simulink model "KP_Nikolaev_v8"  (R2021a)
settings: Solver=VariableStepAuto  StartTime=0.0  StopTime=30  RelTol=0.05
undefined symbols (not defined in the file): D11, Delta
libraries: spsThreePhaseBreakerLib x35, spsSeriesRLCBranchLib x24, spsThreePhaseSeriesRLCLoadLib x22, slrealtimeutilitieslib x14, slrealtimeiplib x13, spsThreePhaseVIMeasurementLib x8, spsExcitationSystemLib x3, spsSynchronousMachinepuStandardLib x3, spsSteamTurbineandGovernorLib x2, spsThreePhaseTransformerTwoWindingsLib x2, spsGroundLib x1, spsHydraulicTurbineandGovernorLib x1
settings Model: Creator=kirill  LastModifiedBy=1
settings SolverCC: AlgebraicLoopSolver=TrustRegion
settings DebuggingCC: UnconnectedInputMsg=none  UnconnectedOutputMsg=none  UnconnectedLineMsg=none  SFMachineParentedDataDiag=warning

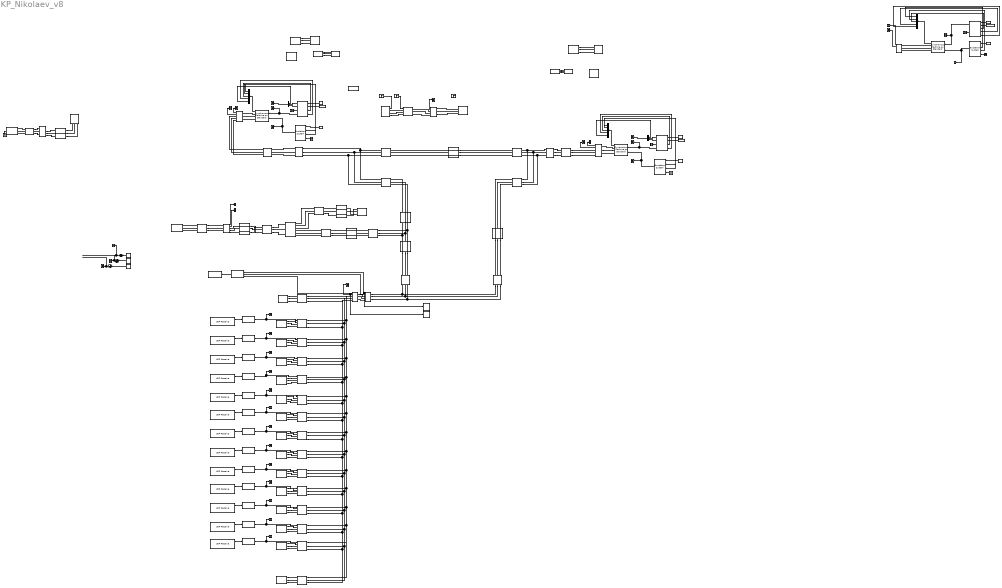
== system KP_Nikolaev_v8 ==
  Breaker0 : spsThreePhaseBreakerLib/Three-Phase Breaker  InitialState=open  SwitchA=on  SwitchB=on  SwitchC=on  SwitchTimes="[1/60  5/60]"  External=off  BreakerResistance=0.01  SnubberResistance=1e6  SnubberCapacitance=inf  Measurements=None
  Breaker{1..13,34} (14 alike) : spsThreePhaseBreakerLib/Three-Phase Breaker  InitialState=closed  SwitchA=on  SwitchB=on  SwitchC=on  SwitchTimes="[1/60  5/60]"  External=on  BreakerResistance=0.01  SnubberResistance=1e6  SnubberCapacitance=inf  Measurements=None
  Breaker{14..32} (19 alike) : spsThreePhaseBreakerLib/Three-Phase Breaker  InitialState=closed  SwitchA=on  SwitchB=on  SwitchC=on  SwitchTimes="[1/60  5/60]"  External=off  BreakerResistance=0.01  SnubberResistance=1e6  SnubberCapacitance=inf  Measurements=None
  Breaker33 : spsThreePhaseBreakerLib/Three-Phase Breaker  InitialState=open  SwitchA=on  SwitchB=on  SwitchC=on  SwitchTimes="[1/60  5/60]"  External=on  BreakerResistance=0.01  SnubberResistance=1e6  SnubberCapacitance=inf  Measurements=None
  Bus Creator1 : BusCreator  Inputs=3
  Bus Creator2 : BusCreator  Inputs=3
  Bus Selector1 : BusSelector  OutputSignals="dq0 components.Stator voltage  vd (pu),dq0 components.Stator voltage  vq (pu),Mechanical.Rotor speed  wm  (pu),Mechanical.Rotor angle deviation  d_theta (rad),Mechanical.Rotor speed deviation  dw (pu)"
  Bus Selector2 : BusSelector  OutputSignals="dq0 components.Stator voltage  vd (pu),dq0 components.Stator voltage  vq (pu),Mechanical.Rotor speed  wm  (pu),Mechanical.Rotor angle deviation  d_theta (rad),Mechanical.Rotor speed deviation  dw (pu)"
  Bus Selector3 : BusSelector  OutputSignals="dq0 components.Stator voltage  vd (pu),dq0 components.Stator voltage  vq (pu),Mechanical.Rotor speed  wm  (pu),Output active power   Peo (pu),Mechanical.Rotor speed deviation  dw (pu)"
  Byte Packing : slrealtimeutilitieslib/Byte Packing  MaskPackedDataType=double  MaskUnpackedDataTypes={'double' 'double' 'double'}  MaskAlignment=1
  Byte Unpacking{,1..11,13} (13 alike) : slrealtimeutilitieslib/Byte Unpacking  MaskUnpackedDataTypes={'double'}  MaskUnpackedDataSizes={[1]}  MaskAlignment=1
      settings: SourceProductBaseCode=XP
  Constant{,1..2,4..5,8} (6 alike) : Constant
  Constant3 : Constant  Value=0.151964
  Constant6 : Constant  Value=0.151964
  Constant7 : Constant  Value=0.90671
  Excitation System : spsExcitationSystemLib/Excitation System  tr=10e-4  reg=[ 200, 0.001 ]  exc=[ 5, 0 ]  tgr=[ 0, 0 ]  damp=[ 0.001, 0.1 ]  sat=[ 0, 0 ]  lim=[ -15, 15, 0 ]  v0=[1,2.93164]
      settings: SourceProductBaseCode=PS
  Excitation System1 : spsExcitationSystemLib/Excitation System  tr=10e-3  reg=[ 19, 0.001 ]  exc=[ 3, 0 ]  tgr=[ 0, 0 ]  damp=[ 0.001, 0.1 ]  sat=[ 0, 0 ]  lim=[ -11.5, 11.5, 0 ]  v0=[1,1.07632]
      settings: SourceProductBaseCode=PS
  Excitation System2 : spsExcitationSystemLib/Excitation System  tr=10e-3  reg=[ 19, 0.001 ]  exc=[ 3, 0 ]  tgr=[ 0, 0 ]  damp=[ 0.001, 0.1 ]  sat=[ 0, 0 ]  lim=[ -11.5, 11.5, 0 ]  v0=[1,1.07632]
      settings: SourceProductBaseCode=PS
  Ground : Ground
  Ground1 : Ground
  Ground2 : Ground
  Ground3 : spsGroundLib/Ground  LConnTagsString=a
  HTG1 : spsHydraulicTurbineandGovernorLib/Hydraulic Turbine and Governor  sm="[ 1  0.77 ]"  gate="[  0.01  0.97518  -0.1  0.1 ]"  reg="[  0.1  0.090 0.005 0.001  1  ]"  hyd="[  0  2.67  ]"  dref=0  po=0.946226
      settings: SourceProductBaseCode=PS
  Scope{1..34} (34 alike) : Scope
  Series RLC Branch{1..3,18..20} (6 alike) : spsSeriesRLCBranchLib/Series RLC Branch  LConnTagsString=__new0  RConnTagsString=__new0  BranchType=RLC  Resistance=12.45  Inductance=70.187e-3  SetiL0=off  InitialCurrent=0  Capacitance=4.07436e-3  Setx0=off  InitialVoltage=0  Measurements=None
  Series RLC Branch{4..6,9..11} (6 alike) : spsSeriesRLCBranchLib/Series RLC Branch  LConnTagsString=__new0  RConnTagsString=__new0  BranchType=RLC  Resistance=6.225  Inductance=35.0935e-3  SetiL0=off  InitialCurrent=0  Capacitance=2.03718e-3  Setx0=off  InitialVoltage=0  Measurements=None
  Series RLC Branch12 : spsSeriesRLCBranchLib/Series RLC Branch  LConnTagsString=__new0  RConnTagsString=__new0  BranchType=RLC  Resistance=9.75  Inductance=70e-3  SetiL0=off  InitialCurrent=0  Capacitance=4.07436e-3  Setx0=off  InitialVoltage=0  Measurements=None
  Series RLC Branch{8,13..14,21} (4 alike) : spsSeriesRLCBranchLib/Series RLC Branch  LConnTagsString=__new0  RConnTagsString=__new0  BranchType=RLC  Resistance=9.75  Inductance=70e-3  SetiL0=off  InitialCurrent=0  Capacitance=4e-3  Setx0=off  InitialVoltage=0  Measurements=None
  Series RLC Branch15 : spsSeriesRLCBranchLib/Series RLC Branch  LConnTagsString=__new0  RConnTagsString=__new0  BranchType=RLC  Resistance=9.25  Inductance=70.187e-3  SetiL0=off  InitialCurrent=0  Capacitance=4.07436e-3  Setx0=off  InitialVoltage=0  Measurements=None
  Series RLC Branch16 : spsSeriesRLCBranchLib/Series RLC Branch  LConnTagsString=__new0  RConnTagsString=__new0  BranchType=RLC  Resistance=9.25  Inductance=70.187e-3  SetiL0=off  InitialCurrent=0  Capacitance=4.07436e-3  Setx0=off  InitialVoltage=0  Measurements=None
  Series RLC Branch17 : spsSeriesRLCBranchLib/Series RLC Branch  LConnTagsString=__new0  RConnTagsString=__new0  BranchType=RLC  Resistance=9.25  Inductance=70.187e-3  SetiL0=off  InitialCurrent=0  Capacitance=4.07436e-3  Setx0=off  InitialVoltage=0  Measurements=None
  Series RLC Branch22 : spsSeriesRLCBranchLib/Series RLC Branch  LConnTagsString=__new0  RConnTagsString=__new0  BranchType=RLC  Resistance=19.5  Inductance=70e-3  SetiL0=off  InitialCurrent=0  Capacitance=4.07436e-3  Setx0=off  InitialVoltage=0  Measurements=None
  Series RLC Branch23 : spsSeriesRLCBranchLib/Series RLC Branch  LConnTagsString=__new0  RConnTagsString=__new0  BranchType=RLC  Resistance=19.5  Inductance=70e-3  SetiL0=off  InitialCurrent=0  Capacitance=4e-3  Setx0=off  InitialVoltage=0  Measurements=None
  Series RLC Branch24 : spsSeriesRLCBranchLib/Series RLC Branch  LConnTagsString=__new0  RConnTagsString=__new0  BranchType=RLC  Resistance=19.5  Inductance=70e-3  SetiL0=off  InitialCurrent=0  Capacitance=4e-3  Setx0=off  InitialVoltage=0  Measurements=None
  Series RLC Branch7 : spsSeriesRLCBranchLib/Series RLC Branch  LConnTagsString=__new0  RConnTagsString=__new0  BranchType=RLC  Resistance=9.75  Inductance=70e-3  SetiL0=off  InitialCurrent=0  Capacitance=4.07436e-3  Setx0=off  InitialVoltage=0  Measurements=None
  Spectrum Analyzer : SpectrumAnalyzer
  Spectrum Analyzer1 : SpectrumAnalyzer
  Steam Turbine and Governor1 : spsSteamTurbineandGovernorLib/Steam Turbine and Governor  gentype=Tandem-compound (single mass)  reg1="[ 5 0.05  0 ]"  reg2="[ 0.001  0.15 ]"  reg3="[ -0.1 0.1  0  10.496]"  N=3000  turb1="[ 0  40 20  2 ]"  turb2="[ 0.5   0.5   0.0  0 ]"  HA="[  1.5498   0.24894  0  0 ]"  KA="[  83.47  42.702  0  0 ]"  DA="[  0.3104  0.05  0  0 ]*8"  ini1=0.173417  ini2=[0.429327,-63.9543]
      settings: SourceProductBaseCode=PS
  Steam Turbine and Governor2 : spsSteamTurbineandGovernorLib/Steam Turbine and Governor  gentype=Tandem-compound (single mass)  reg1="[ 5 0.05  0 ]"  reg2="[ 0.001  0.15 ]"  reg3="[ -0.1 0.1  0  10.496]"  N=3000  turb1="[ 0  40 20  2 ]"  turb2="[ 0.5   0.5   0.0  0 ]"  HA="[  1.5498   0.24894  0  0 ]"  KA="[  83.47  42.702  0  0 ]"  DA="[  0.3104  0.05  0  0 ]*8"  ini1=0.173417  ini2=[0.429327,-63.9543]
      settings: SourceProductBaseCode=PS
  Step : Step  Time=5  SampleTime=0  VectorParams1D=off
  Step1 : Step  Time=7  Before=1  After=0  SampleTime=0  VectorParams1D=off
  Step2 : Step  Time=5  SampleTime=0  VectorParams1D=off
  Sum : Sum  Inputs=|++
  Sum1 : Sum  Inputs=|++
  Sum2 : Sum  Inputs=|++
  Synchronous Machine : spsSynchronousMachinepuStandardLib/Synchronous Machine pu Standard  PresetModel=No  MechanicalLoad=Mechanical power Pm  ShowDetailedParameters=on  RotorType=Salient-pole  Units=per unit standard parameters  MeasurementBus=off  NominalParameters=[25.88e+06 9.785e+03 50]  Reactances1=[ 1.81, 0.3, 0.23, 1.76, 0.65, 0.25, 0.15 ]  Reactances2=[0.8 0.35 0.22 0.59 0.23 0.1]  dAxisTimeConstants=Short-circuit  qAxisTimeConstants=Short-circuit  TimeConstants1="[ 4.4849  0.0681  0.1  ]"  TimeConstants2=[ 8.0, 0.03, 1.0, 0.07 ]  TimeConstants3="[  4.49  0.0681  0.0513  ]"  TimeConstants4=[ 8.0, 0.03, 0.3371, 0.0295 ]  TimeConstants5=[ 1.01, 0.053, 0.1 ]  TimeConstants6=[ 1.3201, 0.023, 1.0, 0.07 ]  TimeConstants7=[0.012 0.003 0.003]  TimeConstants8=[ 1.3201, 0.0231, 0.3371, 0.0295 ]  StatorResistance=0.037875  Mechanical=[0.1028 0.02056 52]  PolePairs=20  InitialConditions=[0 -53.0957 3.14495 3.14495 3.14495 -25.3073 -145.307 94.6927 2.93164]  SetSaturation=on  Saturation=[0.6404,0.7127,0.8441,0.9214,0.9956,1.082,1.19,1.316,1.457;0.7,0.7698,0.8872,0.9466,0.9969,1.046,1.1,1.151,1.201]  LoadFlowParameters=[2 107000000 0 0 0]  TsPowergui=0  TsBlock=-1  IterativeModel=Trapezoidal non iterative  IterativeDiscreteModel=Trapezoidal robust  BusType=swing  Pref=109.0152  Qref=62.94  Qmin=-Inf  Qmax=Inf  PLF=0  QLF=0
      settings: SourceProductBaseCode=PS
  Synchronous Machine1 : spsSynchronousMachinepuStandardLib/Synchronous Machine pu Standard  PresetModel=No  MechanicalLoad=Mechanical power Pm  ShowDetailedParameters=on  RotorType=Round  Units=per unit standard parameters  MeasurementBus=off  NominalParameters=[78.75e+06 7.424e+03 50]  Reactances1=[ 1.915, 0.275, 0.203, 0.82, 0.65, 0.25, 0.15 ]  Reactances2=[1.71 0.172 0.119 0.59 0.23 0.1]  dAxisTimeConstants=Short-circuit  qAxisTimeConstants=Short-circuit  TimeConstants1="[ 4.4849  0.0681  0.1  ]"  TimeConstants2=[ 8.0, 0.03, 1.0, 0.07 ]  TimeConstants3="[  4.49  0.0681  0.0513  ]"  TimeConstants4=[ 8.0, 0.03, 0.3371, 0.0295 ]  TimeConstants5=[ 1.01, 0.053, 0.1 ]  TimeConstants6=[ 1.3201, 0.023, 1.0, 0.07 ]  TimeConstants7=[1.42 0.0908 0.132]  TimeConstants8=[ 1.85, 0.126, 0.212, 0.169 ]  StatorResistance=0.037875  Mechanical=[0.1028 0.02056 1]  PolePairs=20  InitialConditions=[0 -99.9478 0.153639 0.153639 0.153639 -25.3073 -145.307 94.6927 1.07632]  SetSaturation=on  Saturation=[0.6404,0.7127,0.8441,0.9214,0.9956,1.082,1.19,1.316,1.457;0.7,0.7698,0.8872,0.9466,0.9969,1.046,1.1,1.151,1.201]  LoadFlowParameters=[2 7500000 0 0 0]  TsPowergui=0  TsBlock=-1  IterativeModel=Trapezoidal non iterative  IterativeDiscreteModel=Trapezoidal robust  BusType=swing  Pref=2e+06  Qref=1e+06  Qmin=-Inf  Qmax=Inf  PLF=0  QLF=0
      settings: SourceProductBaseCode=PS
  Synchronous Machine2 : spsSynchronousMachinepuStandardLib/Synchronous Machine pu Standard  PresetModel=No  MechanicalLoad=Mechanical power Pm  ShowDetailedParameters=on  RotorType=Round  Units=per unit standard parameters  MeasurementBus=off  NominalParameters=[78.75e+06 7.424e+03 50]  Reactances1=[ 1.915, 0.275, 0.203, 0.82, 0.65, 0.25, 0.15 ]  Reactances2=[1.71 0.172 0.119 0.59 0.23 0.1]  dAxisTimeConstants=Short-circuit  qAxisTimeConstants=Short-circuit  TimeConstants1="[ 4.4849  0.0681  0.1  ]"  TimeConstants2=[ 8.0, 0.03, 1.0, 0.07 ]  TimeConstants3="[  4.49  0.0681  0.0513  ]"  TimeConstants4=[ 8.0, 0.03, 0.3371, 0.0295 ]  TimeConstants5=[ 1.01, 0.053, 0.1 ]  TimeConstants6=[ 1.3201, 0.023, 1.0, 0.07 ]  TimeConstants7=[1.42 0.0908 0.132]  TimeConstants8=[ 1.85, 0.126, 0.212, 0.169 ]  StatorResistance=0.037875  Mechanical=[0.1028 0.02056 1]  PolePairs=20  InitialConditions=[0 -99.9478 0.153639 0.153639 0.153639 -25.3073 -145.307 94.6927 1.07632]  SetSaturation=on  Saturation=[0.6404,0.7127,0.8441,0.9214,0.9956,1.082,1.19,1.316,1.457;0.7,0.7698,0.8872,0.9466,0.9969,1.046,1.1,1.151,1.201]  LoadFlowParameters=[2 7500000 0 0 0]  TsPowergui=0  TsBlock=-1  IterativeModel=Trapezoidal non iterative  IterativeDiscreteModel=Trapezoidal robust  BusType=swing  Pref=2e+06  Qref=1e+06  Qmin=-Inf  Qmax=Inf  PLF=0  QLF=0
      settings: SourceProductBaseCode=PS
  T1 : spsThreePhaseTransformerInductanceMatrixTypeThreeWindingsLib/Three-Phase Transformer Inductance Matrix Type (Three Windings)  CoreType=Three single-phase cores  Winding1Connection=Y  Winding2Connection=Delta (D11)  Winding3Connection=Delta (D11)  AutoTransformer=off  Measurements=None  NominalPower="[133e6,  50]"  VLLnom="[330e3,  230e3,  38.5e3]"  WindingResistances="[0.005,  0.005, 0.005]"  NoLoadIexcPos=0.06  NoLoadPlossPos=50e3  ShortCircuitReactancePos="[0.087,  0.166,  0.067]"  ShortCircuitReactancePosAuto="[0.087,  0.166,  0.067]"  NoLoadIexcZero=100  NoLoadPlossZero=133e6*1/100  ShortCircuitReactanceZero=[0.1, 0.2, 0.3 ]  ShortCircuitReactanceZeroAuto=[0.1, 0.2, 0.3 ]  X12ZeroMeasuredWithW3Delta=off
      settings: SourceProductBaseCode=PS
  Terminator : Terminator
  Terminator1 : Terminator
  Terminator2 : Terminator
  Three-Phase Measurement 1 : spsThreePhaseVIMeasurementLib/Three-Phase V-I Measurement  VoltageMeasurement=phase-to-ground  SetLabelV=off  LabelV=Vabc  Vpu=off  VpuLL=off  CurrentMeasurement=yes  SetLabelI=off  LabelI=Iabc  Ipu=off  Pbase=100e6  Vbase=115e3  OutputType=Complex  PhasorSimulation=off  PSBequivalent=0
  Three-Phase Measurement 2 : spsThreePhaseVIMeasurementLib/Three-Phase V-I Measurement  VoltageMeasurement=phase-to-phase  SetLabelV=off  LabelV=Vabc  Vpu=off  VpuLL=off  CurrentMeasurement=yes  SetLabelI=off  LabelI=Iabc  Ipu=off  Pbase=100e6  Vbase=500e3  OutputType=Complex  PhasorSimulation=off  PSBequivalent=0
  Three-Phase Measurement 4 : spsThreePhaseVIMeasurementLib/Three-Phase V-I Measurement  VoltageMeasurement=phase-to-ground  SetLabelV=off  LabelV=Vabc  Vpu=off  VpuLL=off  CurrentMeasurement=yes  SetLabelI=off  LabelI=Iabc  Ipu=off  Pbase=100e6  Vbase=115e3  OutputType=Complex  PhasorSimulation=off  PSBequivalent=0
  Three-Phase Measurement 9 : spsThreePhaseVIMeasurementLib/Three-Phase V-I Measurement  VoltageMeasurement=phase-to-phase  SetLabelV=off  LabelV=Vabc  Vpu=off  VpuLL=off  CurrentMeasurement=yes  SetLabelI=off  LabelI=Iabc  Ipu=off  Pbase=100e6  Vbase=500e3  OutputType=Complex  PhasorSimulation=off  PSBequivalent=0
  Three-Phase RL Load0 : spsThreePhaseSeriesRLCLoadLib/Three-Phase Series RLC Load  LConnTagsString=A|B|C  Configuration=Y (grounded)  NominalVoltage=230000  Vabc=[1e3 1e3 1e3]  Vabcp=[1e3 1e3 1e3]  NominalFrequency=50  UnbalancedPower=off  ActivePower=78.5225e+06  InductivePower=33.4873e+06  CapacitivePower=500  Pabc=[10e3 9e3 11e3]  QLabc=[100 90 110]  QCabc=[100 90 110]  Pabcp=[10e3 9e3 11e3]  QLabcp=[100 90 110]  QCabcp=[100 90 110]  Measurements=None  LoadType=constant PQ
  Three-Phase RL Load{1..11} (11 alike) : spsThreePhaseSeriesRLCLoadLib/Three-Phase Series RLC Load  LConnTagsString=A|B|C  Configuration=Y (grounded)  NominalVoltage=230000  Vabc=[1e3 1e3 1e3]  Vabcp=[1e3 1e3 1e3]  NominalFrequency=50  UnbalancedPower=off  ActivePower=8.144e+06  InductivePower=3.47264e+06  CapacitivePower=50  Pabc=[10e3 9e3 11e3]  QLabc=[100 90 110]  QCabc=[100 90 110]  Pabcp=[10e3 9e3 11e3]  QLabcp=[100 90 110]  QCabcp=[100 90 110]  Measurements=None  LoadType=constant PQ
  Three-Phase RL Load12 : spsThreePhaseSeriesRLCLoadLib/Three-Phase Series RLC Load  LConnTagsString=A|B|C  Configuration=Y (grounded)  NominalVoltage=230000  Vabc=[1e3 1e3 1e3]  Vabcp=[1e3 1e3 1e3]  NominalFrequency=50  UnbalancedPower=off  ActivePower=17.948e+06  InductivePower=7.6532e+06  CapacitivePower=100  Pabc=[10e3 9e3 11e3]  QLabc=[100 90 110]  QCabc=[100 90 110]  Pabcp=[10e3 9e3 11e3]  QLabcp=[100 90 110]  QCabcp=[100 90 110]  Measurements=None  LoadType=constant PQ
  Three-Phase RL Load13 : spsThreePhaseSeriesRLCLoadLib/Three-Phase Series RLC Load  LConnTagsString=A|B|C  Configuration=Y (grounded)  NominalVoltage=230000  Vabc=[1e3 1e3 1e3]  Vabcp=[1e3 1e3 1e3]  NominalFrequency=50  UnbalancedPower=off  ActivePower=17.948e+06  InductivePower=7.6532e+06  CapacitivePower=100  Pabc=[10e3 9e3 11e3]  QLabc=[100 90 110]  QCabc=[100 90 110]  Pabcp=[10e3 9e3 11e3]  QLabcp=[100 90 110]  QCabcp=[100 90 110]  Measurements=None  LoadType=constant PQ
  Three-Phase RL Load14 : spsThreePhaseSeriesRLCLoadLib/Three-Phase Series RLC Load  LConnTagsString=A|B|C  Configuration=Y (grounded)  NominalVoltage=10500  Vabc=[1e3 1e3 1e3]  Vabcp=[1e3 1e3 1e3]  NominalFrequency=50  UnbalancedPower=off  ActivePower=4500  InductivePower=0  CapacitivePower=0  Pabc=[10e3 9e3 11e3]  QLabc=[100 90 110]  QCabc=[100 90 110]  Pabcp=[10e3 9e3 11e3]  QLabcp=[100 90 110]  QCabcp=[100 90 110]  Measurements=None  LoadType=constant PQ
  Three-Phase RL Load15 : spsThreePhaseSeriesRLCLoadLib/Three-Phase Series RLC Load  LConnTagsString=A|B|C  Configuration=Y (grounded)  NominalVoltage=230000  Vabc=[1e3 1e3 1e3]  Vabcp=[1e3 1e3 1e3]  NominalFrequency=50  UnbalancedPower=off  ActivePower=98.714e+06  InductivePower=42.0926e+06  CapacitivePower=1000  Pabc=[10e3 9e3 11e3]  QLabc=[100 90 110]  QCabc=[100 90 110]  Pabcp=[10e3 9e3 11e3]  QLabcp=[100 90 110]  QCabcp=[100 90 110]  Measurements=None  LoadType=constant PQ
  Three-Phase RL Load16 : spsThreePhaseSeriesRLCLoadLib/Three-Phase Series RLC Load  LConnTagsString=A|B|C  Configuration=Y (grounded)  NominalVoltage=10500  Vabc=[1e3 1e3 1e3]  Vabcp=[1e3 1e3 1e3]  NominalFrequency=50  UnbalancedPower=off  ActivePower=4500  InductivePower=0  CapacitivePower=0  Pabc=[10e3 9e3 11e3]  QLabc=[100 90 110]  QCabc=[100 90 110]  Pabcp=[10e3 9e3 11e3]  QLabcp=[100 90 110]  QCabcp=[100 90 110]  Measurements=None  LoadType=constant PQ
  Three-Phase RL Load17 : spsThreePhaseSeriesRLCLoadLib/Three-Phase Series RLC Load  LConnTagsString=A|B|C  Configuration=Y (grounded)  NominalVoltage=10500  Vabc=[1e3 1e3 1e3]  Vabcp=[1e3 1e3 1e3]  NominalFrequency=50  UnbalancedPower=off  ActivePower=1.75e+06  InductivePower=1e+06  CapacitivePower=100  Pabc=[10e3 9e3 11e3]  QLabc=[100 90 110]  QCabc=[100 90 110]  Pabcp=[10e3 9e3 11e3]  QLabcp=[100 90 110]  QCabcp=[100 90 110]  Measurements=None  LoadType=constant PQ
  Three-Phase RL Load18 : spsThreePhaseSeriesRLCLoadLib/Three-Phase Series RLC Load  LConnTagsString=A|B|C  Configuration=Y (grounded)  NominalVoltage=10500  Vabc=[1e3 1e3 1e3]  Vabcp=[1e3 1e3 1e3]  NominalFrequency=50  UnbalancedPower=off  ActivePower=3.25e+06  InductivePower=1.875e+06  CapacitivePower=100  Pabc=[10e3 9e3 11e3]  QLabc=[100 90 110]  QCabc=[100 90 110]  Pabcp=[10e3 9e3 11e3]  QLabcp=[100 90 110]  QCabcp=[100 90 110]  Measurements=None  LoadType=constant PQ
  Three-Phase RL Load19 : spsThreePhaseSeriesRLCLoadLib/Three-Phase Series RLC Load  LConnTagsString=A|B|C  Configuration=Y (grounded)  NominalVoltage=10500  Vabc=[1e3 1e3 1e3]  Vabcp=[1e3 1e3 1e3]  NominalFrequency=50  UnbalancedPower=off  ActivePower=1.75e+06  InductivePower=1e+06  CapacitivePower=100  Pabc=[10e3 9e3 11e3]  QLabc=[100 90 110]  QCabc=[100 90 110]  Pabcp=[10e3 9e3 11e3]  QLabcp=[100 90 110]  QCabcp=[100 90 110]  Measurements=None  LoadType=constant PQ
  Three-Phase RL Load20 : spsThreePhaseSeriesRLCLoadLib/Three-Phase Series RLC Load  LConnTagsString=A|B|C  Configuration=Y (grounded)  NominalVoltage=10500  Vabc=[1e3 1e3 1e3]  Vabcp=[1e3 1e3 1e3]  NominalFrequency=50  UnbalancedPower=off  ActivePower=3.25e+06  InductivePower=1.875e+06  CapacitivePower=100  Pabc=[10e3 9e3 11e3]  QLabc=[100 90 110]  QCabc=[100 90 110]  Pabcp=[10e3 9e3 11e3]  QLabcp=[100 90 110]  QCabcp=[100 90 110]  Measurements=None  LoadType=constant PQ
  Three-Phase RL Load21 : spsThreePhaseSeriesRLCLoadLib/Three-Phase Series RLC Load  LConnTagsString=A|B|C  Configuration=Y (grounded)  NominalVoltage=38.5e3  Vabc=[1e3 1e3 1e3]  Vabcp=[1e3 1e3 1e3]  NominalFrequency=50  UnbalancedPower=off  ActivePower=13.65e+06  InductivePower=7.875e+06  CapacitivePower=100  Pabc=[10e3 9e3 11e3]  QLabc=[100 90 110]  QCabc=[100 90 110]  Pabcp=[10e3 9e3 11e3]  QLabcp=[100 90 110]  QCabcp=[100 90 110]  Measurements=None  LoadType=constant PQ
  Three-Phase Transformer (Two Windings)1 : spsThreePhaseTransformerTwoWindingsLib/Three-Phase Transformer (Two Windings)  Winding1Connection=Y  Winding2Connection=Delta (D11)  CoreType=Three single-phase transformers  SetSaturation=off  Hysteresis=off  DataFile='hysteresis'  SetInitialFlux=off  Measurements=None  UNITS=SI  NominalPower=[ 80e6 , 50 ]  Winding1=[10500 0.00882 0.001123]  Winding2=[2.42e+05 11.616 1.479]  Rm=2205  Lm=7.0187  L0=0.5  Saturation=[0 0;4.6657 32.747;1944 41.48]  InitialFluxes=[ 0.8 , -0.8 , 0.7 ]  BreakLoop=on  DiscreteSolver=Trapezoidal iterative  DataType=on  TransfoNumber=1
  Three-Phase Transformer (Two Windings)2 : spsThreePhaseTransformerTwoWindingsLib/Three-Phase Transformer (Two Windings)  Winding1Connection=Y  Winding2Connection=Delta (D11)  CoreType=Three single-phase transformers  SetSaturation=off  Hysteresis=off  DataFile='hysteresis'  SetInitialFlux=off  Measurements=None  UNITS=SI  NominalPower=[ 80e6 , 50 ]  Winding1=[10500 0.00882 0.001123]  Winding2=[2.42e+05 11.616 1.479]  Rm=2205  Lm=7.0187  L0=0.5  Saturation=[0 0;4.6657 32.747;1944 41.48]  InitialFluxes=[ 0.8 , -0.8 , 0.7 ]  BreakLoop=on  DiscreteSolver=Trapezoidal iterative  DataType=on  TransfoNumber=1
  Three-Phase V-I Measurement1 : spsThreePhaseVIMeasurementLib/Three-Phase V-I Measurement  VoltageMeasurement=phase-to-phase  SetLabelV=off  LabelV=Vabc  Vpu=off  VpuLL=off  CurrentMeasurement=yes  SetLabelI=off  LabelI=Iabc  Ipu=off  Pbase=100e6  Vbase=10.5e3  OutputType=Complex  PhasorSimulation=off  PSBequivalent=0
  Three-Phase V-I Measurement2 : spsThreePhaseVIMeasurementLib/Three-Phase V-I Measurement  VoltageMeasurement=phase-to-phase  SetLabelV=off  LabelV=Vabc  Vpu=off  VpuLL=off  CurrentMeasurement=yes  SetLabelI=off  LabelI=Iabc  Ipu=off  Pbase=100e6  Vbase=10.5e3  OutputType=Complex  PhasorSimulation=off  PSBequivalent=0
  Three-Phase V-I Measurement3 : spsThreePhaseVIMeasurementLib/Three-Phase V-I Measurement  VoltageMeasurement=phase-to-phase  SetLabelV=off  LabelV=Vabc  Vpu=off  VpuLL=off  CurrentMeasurement=yes  SetLabelI=off  LabelI=Iabc  Ipu=off  Pbase=100e6  Vbase=500e3  OutputType=Complex  PhasorSimulation=off  PSBequivalent=0
  Three-Phase V-I Measurement4 : spsThreePhaseVIMeasurementLib/Three-Phase V-I Measurement  VoltageMeasurement=phase-to-ground  SetLabelV=off  LabelV=Vabc  Vpu=off  VpuLL=off  CurrentMeasurement=yes  SetLabelI=off  LabelI=Iabc  Ipu=off  Pbase=100e6  Vbase=500e3  OutputType=Complex  PhasorSimulation=off  PSBequivalent=0
  Three-Phase Fault : spsThreePhaseFaultLib/Three-Phase Fault  InitialStates=0  FaultA=on  FaultB=on  FaultC=on  GroundFault=on  SwitchTimes="[1/60  5/60]"  External=on  SwitchStatus=NaN  FaultResistance=0.001  GroundResistance=0.01  SnubberResistance=1e6  SnubberCapacitance=inf  Measurements=None
  Three-Phase Programmable Voltage Source4 : spsThreePhaseProgrammableVoltageSourceLib/Three-Phase Programmable Voltage Source  PositiveSequence="[230000  0 50]"  VariationEntity=None  VariationType=Table of time-amplitude pairs  VariationTypeAlt=Step  VariationStep=0.5  VariationRate=10  VariationMagnitude=0.3  VariationFrequency=2  VariationTiming=[1 2]  VariationPhaseA=off  Amplitudes=[1 0.8 1.2 1.0]  TimeValues=[0 0.1 0.15 0.2]  HarmonicGeneration=off  HarmonicA=[3 0.2 -25 0]  HarmonicB=[2 0.15 35 2]  Timing="[0.05  3]"  BusType=swing  Pref=0  Qref=0  Qmin=-inf  Qmax=inf
  Three-Phase Series RLC Branch4 : spsThreePhaseSeriesRLCBranchLib/Three-Phase Series RLC Branch  LConnTagsString=A|B|C  RConnTagsString=A|B|C  BranchType=RL  Resistance=0.005  Inductance=1e-06  Capacitance=1e-6  Measurements=None
  Three-Phase Source1 : spsThreePhaseSourceLib/Three-Phase Source  InternalConnection=Yg  VoltagePhases=off  Voltage=245375  PhaseAngle=0  Voltage_phases=[25e3 25e3 25e3]/sqrt(3)  PhaseAngles_phases=[0 -120 +120]  Frequency=50  NonIdealSource=on  SpecifyImpedance=off  Resistance=0.005  Inductance=1e-06  ShortCircuitLevel=100e6  BaseVoltage=190525.5888  XRratio=7  BusType=PV  Pref=125.714e6  Qref=15e6  Prefabc=[10e3, 10e3, 10e3]  Qrefabc=[0, 0, 0]  Qmin=0  Qmax=15e6
  UDP Receive1 : slrealtimeiplib/UDP Receive  useHostTargetConn=on  ipAddress='localhost'  localPort=9002  rcvWidth=8  rcvFmAny=on  fmAddress=10.10.10.10  sampleTime=10e-5
      settings: SourceProductBaseCode=XP
  UDP Receive10 : slrealtimeiplib/UDP Receive  useHostTargetConn=on  ipAddress='localhost'  localPort=9011  rcvWidth=8  rcvFmAny=on  fmAddress=10.10.10.10  sampleTime=10e-5
      settings: SourceProductBaseCode=XP
  UDP Receive11 : slrealtimeiplib/UDP Receive  useHostTargetConn=on  ipAddress='localhost'  localPort=9012  rcvWidth=8  rcvFmAny=on  fmAddress=10.10.10.10  sampleTime=10e-5
      settings: SourceProductBaseCode=XP
  UDP Receive12 : slrealtimeiplib/UDP Receive  useHostTargetConn=on  ipAddress='localhost'  localPort=9013  rcvWidth=8  rcvFmAny=on  fmAddress=10.10.10.10  sampleTime=10e-5
      settings: SourceProductBaseCode=XP
  UDP Receive14 : slrealtimeiplib/UDP Receive  useHostTargetConn=on  ipAddress='localhost'  localPort=9001  rcvWidth=8  rcvFmAny=on  fmAddress=10.10.10.10  sampleTime=10e-5
      settings: SourceProductBaseCode=XP
  UDP Receive2 : slrealtimeiplib/UDP Receive  useHostTargetConn=on  ipAddress='localhost'  localPort=9003  rcvWidth=8  rcvFmAny=on  fmAddress=10.10.10.10  sampleTime=10e-5
      settings: SourceProductBaseCode=XP
  UDP Receive3 : slrealtimeiplib/UDP Receive  useHostTargetConn=on  ipAddress='localhost'  localPort=9004  rcvWidth=8  rcvFmAny=on  fmAddress=10.10.10.10  sampleTime=10e-5
      settings: SourceProductBaseCode=XP
  UDP Receive4 : slrealtimeiplib/UDP Receive  useHostTargetConn=on  ipAddress='localhost'  localPort=9005  rcvWidth=8  rcvFmAny=on  fmAddress=10.10.10.10  sampleTime=10e-5
      settings: SourceProductBaseCode=XP
  UDP Receive5 : slrealtimeiplib/UDP Receive  useHostTargetConn=on  ipAddress='localhost'  localPort=9006  rcvWidth=8  rcvFmAny=on  fmAddress=10.10.10.10  sampleTime=10e-5
      settings: SourceProductBaseCode=XP
  UDP Receive6 : slrealtimeiplib/UDP Receive  useHostTargetConn=on  ipAddress='localhost'  localPort=9007  rcvWidth=8  rcvFmAny=on  fmAddress=10.10.10.10  sampleTime=10e-5
      settings: SourceProductBaseCode=XP
  UDP Receive7 : slrealtimeiplib/UDP Receive  useHostTargetConn=on  ipAddress='localhost'  localPort=9008  rcvWidth=8  rcvFmAny=on  fmAddress=10.10.10.10  sampleTime=10e-5
      settings: SourceProductBaseCode=XP
  UDP Receive8 : slrealtimeiplib/UDP Receive  useHostTargetConn=on  ipAddress='localhost'  localPort=9009  rcvWidth=8  rcvFmAny=on  fmAddress=10.10.10.10  sampleTime=10e-5
      settings: SourceProductBaseCode=XP
  UDP Receive9 : slrealtimeiplib/UDP Receive  useHostTargetConn=on  ipAddress='localhost'  localPort=9010  rcvWidth=8  rcvFmAny=on  fmAddress=10.10.10.10  sampleTime=10e-5
      settings: SourceProductBaseCode=XP
  UDP Send : dspnetwork/UDP Send  remoteURL='localhost'  remotePort=9090  localURL='0.0.0.0'  localPortSource=Automatically determine  localPort=-1  sendBufferSize=24  sampletime=-1  blockPlatform=[]  separateLengthPort=0
  Uniform Random Number : UniformRandomNumber  Minimum=-10000  Maximum=10000  SampleTime=10e-5  VectorParams1D=off
  Uniform Random Number1 : UniformRandomNumber  Minimum=-10  Maximum=10  SampleTime=10e-5
  Uniform Random Number2 : UniformRandomNumber  Minimum=-5000  Maximum=5000  SampleTime=0.1
  powergui : spspowerguiLib/powergui  Priority=1  SimulationMode=Discrete  SampleTime=0.00025  frequency=60  Iterations=50  frequencyindice=0  Pbase=100e6  ErrMax=1e-4  UnitsV=kV  UnitsW=MW  buscounter=0  FunctionMessages=off  echomessages=off  EnableUseOfTLC=off  CurrentSourceSwitches=off  DisableSnubberDevices=off  DisableRonSwitches=off  DisableVfSwitches=off  DisplayEquations=off  AutomaticDiscreteSolvers=off  SolverType=Tustin/Backward Euler (TBE)  Interpol=off  ExternalGateDelay=off  methode=off  Ts=100  x0status=blocks  SPID=on  SwTol=0  HookPort=off  NonlinearTolerance=1e-4  nMaxIteration=100  ContinueOnMaxIteration=off  RestoreLinks=warning  ResistiveCurrentMeasurement=off  Frange=[0:2:500]  Ylog=off  Xlog=on  ShowGrid=off  save=off  variable=ZData  structure=0  ZoomFFT=off  StartTime=0.0  cycles=1  DisplayStyle=1  fundamental=60  FreqAxis=off  MaxFrequency=1000  frequencyindicesteady=1  RmsSteady=1  display=off
  wires:
  Bus Selector1/3 -> Steam Turbine and Governor1/3  "<Rotor speed  wm  (pu)>"
  Ground1/1 -> Excitation System1/4
  Steam Turbine and Governor1/2 -> Bus Creator2/3
  Synchronous Machine1/1 -> Bus Selector1/1
  Bus Selector1/1 -> Excitation System1/2  "<Stator voltage  vd (pu)>"
  Steam Turbine and Governor1/1 -> Bus Creator2/2
  Three-Phase V-I Measurement2/1 -> Scope5/1
  Bus Creator2/1 -> Scope7/1
  Excitation System1/1 -> Synchronous Machine1/2, Scope10/1
  Constant2/1 -> Steam Turbine and Governor1/1
  Constant3/1 -> Steam Turbine and Governor1/2
  Bus Selector1/5 -> Bus Creator2/1  "<Rotor speed deviation  dw (pu)>"
  Steam Turbine and Governor1/3 -> Terminator1/1
  Bus Selector1/4 -> Steam Turbine and Governor1/4  "<Rotor angle deviation  d_theta (rad)>"
  Three-Phase V-I Measurement2/2 -> Scope8/1
  Steam Turbine and Governor1/4 -> Synchronous Machine1/1, Scope9/1
  Constant1/1 -> Excitation System1/1
  Bus Selector1/2 -> Excitation System1/3  "<Stator voltage  vq (pu)>"
  Bus Selector2/3 -> Steam Turbine and Governor2/3  "<Rotor speed  wm  (pu)>"
  Ground2/1 -> Excitation System2/4
  Steam Turbine and Governor2/2 -> Bus Creator1/3
  Synchronous Machine2/1 -> Bus Selector2/1
  Bus Selector2/1 -> Excitation System2/2  "<Stator voltage  vd (pu)>"
  Steam Turbine and Governor2/1 -> Bus Creator1/2
  Three-Phase V-I Measurement1/1 -> Scope2/1
  Bus Creator1/1 -> Scope3/1
  Excitation System2/1 -> Synchronous Machine2/2, Scope1/1
  Constant5/1 -> Steam Turbine and Governor2/1
  Constant6/1 -> Steam Turbine and Governor2/2
  Bus Selector2/5 -> Bus Creator1/1  "<Rotor speed deviation  dw (pu)>"
  Steam Turbine and Governor2/3 -> Terminator2/1
  Bus Selector2/4 -> Steam Turbine and Governor2/4  "<Rotor angle deviation  d_theta (rad)>"
  Three-Phase V-I Measurement1/2 -> Scope4/1
  Steam Turbine and Governor2/4 -> Synchronous Machine2/1, Scope6/1
  Constant4/1 -> Excitation System2/1
  Bus Selector2/2 -> Excitation System2/3  "<Stator voltage  vq (pu)>"
  UDP Receive3/1 -> Byte Unpacking2/1
  Byte Unpacking2/1 -> Scope23/1, Breaker4/1
  UDP Receive14/1 -> Byte Unpacking13/1
  UDP Receive9/1 -> Byte Unpacking8/1
  Byte Unpacking7/1 -> Breaker9/1, Scope28/1
  Byte Unpacking13/1 -> Breaker1/1, Scope14/1
  UDP Receive6/1 -> Byte Unpacking5/1
  UDP Receive7/1 -> Byte Unpacking6/1
  Byte Unpacking4/1 -> Breaker6/1, Scope25/1
  Byte Unpacking11/1 -> Breaker13/1, Scope12/1
  UDP Receive1/1 -> Byte Unpacking/1
  Byte Unpacking3/1 -> Breaker5/1, Scope24/1
  Byte Unpacking1/1 -> Breaker3/1, Scope22/1
  UDP Receive5/1 -> Byte Unpacking4/1
  UDP Receive4/1 -> Byte Unpacking3/1
  UDP Receive2/1 -> Byte Unpacking1/1
  UDP Receive8/1 -> Byte Unpacking7/1
  Byte Unpacking8/1 -> Breaker10/1, Scope29/1
  Byte Unpacking10/1 -> Breaker12/1, Scope11/1
  UDP Receive10/1 -> Byte Unpacking9/1
  Byte Unpacking5/1 -> Breaker7/1, Scope26/1
  Byte Unpacking9/1 -> Breaker11/1, Scope30/1
  Byte Unpacking6/1 -> Breaker8/1, Scope27/1
  UDP Receive11/1 -> Byte Unpacking10/1
  UDP Receive12/1 -> Byte Unpacking11/1
  Byte Unpacking/1 -> Breaker2/1, Scope19/1
  Byte Packing/1 -> UDP Send/1
  Three-Phase Measurement 4/2 -> Byte Packing/2
  Three-Phase Measurement 1/1 -> Byte Packing/3
  Three-Phase Measurement 1/2 -> Spectrum Analyzer1/1, Scope13/1
  Three-Phase Measurement 9/2 -> Scope15/1
  Three-Phase Measurement 9/1 -> Scope21/1
  Step2/1 -> Three-Phase Fault/1
  Three-Phase V-I Measurement3/2 -> Scope16/1
  Step/1 -> Breaker33/1
  Uniform Random Number2/1 -> Sum2/1
  Sum/1 -> Scope31/1
  Sum1/1 -> Scope18/1
  Sum2/1 -> Scope17/1
  ? -> Sum2/2
  ? -> Sum/2
  Uniform Random Number/1 -> Sum/1
  Uniform Random Number1/1 -> Sum1/1
  ? -> Sum1/2
  Three-Phase Measurement 2/1 -> Scope32/1
  Bus Selector3/3 -> HTG1/3  "<Rotor speed  wm  (pu)>"
  HTG1/1 -> Synchronous Machine/1, Scope33/1
  HTG1/2 -> Terminator/1
  Synchronous Machine/1 -> Bus Selector3/1
  Constant8/1 -> Excitation System/1
  Ground/1 -> Excitation System/4
  Bus Selector3/5 -> HTG1/5  "<Rotor speed deviation  dw (pu)>"
  Constant/1 -> HTG1/1
  Bus Selector3/4 -> HTG1/4  "<Output active power   Peo (pu)>"
  Three-Phase Measurement 2/2 -> Scope20/1
  Excitation System/1 -> Scope34/1, Synchronous Machine/2
  Bus Selector3/2 -> Excitation System/3  "<Stator voltage  vq (pu)>"
  Bus Selector3/1 -> Excitation System/2  "<Stator voltage  vd (pu)>"
  Constant7/1 -> HTG1/2
  Three-Phase Measurement 4/1 -> Spectrum Analyzer/1, Byte Packing/1
  connections:
  Three-Phase RL Load0/LConn2 -- Breaker0/LConn2
  Three-Phase RL Load0/LConn1 -- Breaker0/LConn1
  Three-Phase RL Load0/LConn3 -- Breaker0/LConn3
  Breaker1/RConn3 -- Three-Phase Measurement 1/RConn3 -- Breaker0/RConn3 -- Breaker3/RConn3 -- Breaker4/RConn3 -- Breaker5/RConn3 -- Breaker6/RConn3 -- Breaker7/RConn3 -- Breaker8/RConn3 -- Breaker9/RConn3 -- Breaker10/RConn3 -- Breaker11/RConn3 -- Breaker15/RConn3 -- Breaker13/RConn3 -- Breaker12/RConn3 -- Breaker2/RConn3
  Breaker1/RConn2 -- Breaker0/RConn2 -- Three-Phase Measurement 1/RConn2 -- Breaker2/RConn2 -- Breaker3/RConn2 -- Breaker4/RConn2 -- Breaker5/RConn2 -- Breaker6/RConn2 -- Breaker7/RConn2 -- Breaker8/RConn2 -- Breaker9/RConn2 -- Breaker10/RConn2 -- Breaker11/RConn2 -- Breaker15/RConn2 -- Breaker13/RConn2 -- Breaker12/RConn2
  Breaker15/RConn1 -- Breaker13/RConn1 -- Breaker12/RConn1 -- Breaker11/RConn1 -- Breaker10/RConn1 -- Breaker9/RConn1 -- Breaker8/RConn1 -- Breaker7/RConn1 -- Breaker6/RConn1 -- Breaker5/RConn1 -- Breaker4/RConn1 -- Breaker3/RConn1 -- Breaker0/RConn1 -- Three-Phase Measurement 1/RConn1 -- Breaker1/RConn1 -- Breaker2/RConn1
  Three-Phase RL Load2/LConn3 -- Breaker2/LConn3
  Three-Phase RL Load2/LConn2 -- Breaker2/LConn2
  Three-Phase RL Load2/LConn1 -- Breaker2/LConn1
  Three-Phase RL Load3/LConn2 -- Breaker3/LConn2
  Three-Phase RL Load3/LConn3 -- Breaker3/LConn3
  Three-Phase RL Load3/LConn1 -- Breaker3/LConn1
  Three-Phase RL Load4/LConn3 -- Breaker4/LConn3
  Three-Phase RL Load4/LConn1 -- Breaker4/LConn1
  Three-Phase RL Load5/LConn2 -- Breaker5/LConn2
  Three-Phase RL Load4/LConn2 -- Breaker4/LConn2
  Three-Phase RL Load5/LConn3 -- Breaker5/LConn3
  Three-Phase RL Load5/LConn1 -- Breaker5/LConn1
  Three-Phase RL Load9/LConn3 -- Breaker9/LConn3
  Three-Phase RL Load6/LConn1 -- Breaker6/LConn1
  Three-Phase RL Load7/LConn2 -- Breaker7/LConn2
  Three-Phase RL Load8/LConn1 -- Breaker8/LConn1
  Three-Phase RL Load9/LConn2 -- Breaker9/LConn2
  Three-Phase RL Load7/LConn3 -- Breaker7/LConn3
  Three-Phase RL Load9/LConn1 -- Breaker9/LConn1
  Three-Phase RL Load6/LConn2 -- Breaker6/LConn2
  Three-Phase RL Load6/LConn3 -- Breaker6/LConn3
  Three-Phase RL Load7/LConn1 -- Breaker7/LConn1
  Three-Phase RL Load8/LConn3 -- Breaker8/LConn3
  Three-Phase RL Load8/LConn2 -- Breaker8/LConn2
  Three-Phase RL Load10/LConn1 -- Breaker10/LConn1
  Three-Phase RL Load11/LConn2 -- Breaker11/LConn2
  Three-Phase RL Load11/LConn3 -- Breaker11/LConn3
  Three-Phase RL Load10/LConn2 -- Breaker10/LConn2
  Three-Phase RL Load10/LConn3 -- Breaker10/LConn3
  Three-Phase RL Load11/LConn1 -- Breaker11/LConn1
  Three-Phase RL Load12/LConn1 -- Breaker12/LConn1
  Three-Phase RL Load12/LConn2 -- Breaker12/LConn2
  Three-Phase RL Load12/LConn3 -- Breaker12/LConn3
  Three-Phase RL Load13/LConn3 -- Breaker13/LConn3
  Three-Phase RL Load13/LConn2 -- Breaker13/LConn2
  Three-Phase RL Load13/LConn1 -- Breaker13/LConn1
  Three-Phase RL Load15/LConn1 -- Breaker15/LConn1
  Three-Phase RL Load15/LConn3 -- Breaker15/LConn3
  Three-Phase RL Load15/LConn2 -- Breaker15/LConn2
  Three-Phase RL Load1/LConn1 -- Breaker1/LConn1
  Three-Phase RL Load1/LConn2 -- Breaker1/LConn2
  Three-Phase RL Load1/LConn3 -- Breaker1/LConn3
  Breaker17/LConn1 -- Three-Phase Transformer (Two Windings)2/RConn1 -- Breaker16/LConn1
  Breaker17/LConn2 -- Three-Phase Transformer (Two Windings)2/RConn2 -- Breaker16/LConn2
  Breaker17/LConn3 -- Three-Phase Transformer (Two Windings)2/RConn3 -- Breaker16/LConn3
  Breaker18/RConn3 -- Three-Phase Transformer (Two Windings)1/RConn3 -- Breaker19/RConn3
  Breaker18/RConn2 -- Three-Phase Transformer (Two Windings)1/RConn2 -- Breaker19/RConn2
  Breaker18/RConn1 -- Three-Phase Transformer (Two Windings)1/RConn1 -- Breaker19/RConn1
  Three-Phase V-I Measurement2/LConn2 -- Synchronous Machine1/RConn2
  Synchronous Machine1/RConn1 -- Three-Phase V-I Measurement2/LConn1
  Synchronous Machine1/RConn3 -- Three-Phase V-I Measurement2/LConn3
  Synchronous Machine2/RConn2 -- Three-Phase V-I Measurement1/LConn2
  Synchronous Machine2/RConn1 -- Three-Phase V-I Measurement1/LConn1
  Synchronous Machine2/RConn3 -- Three-Phase V-I Measurement1/LConn3
  Three-Phase RL Load18/LConn1 -- Breaker22/LConn1
  Three-Phase RL Load18/LConn2 -- Breaker22/LConn2
  Three-Phase RL Load17/LConn1 -- Breaker14/RConn1
  Three-Phase RL Load17/LConn3 -- Breaker14/RConn3
  Three-Phase RL Load17/LConn2 -- Breaker14/RConn2
  Three-Phase RL Load18/LConn3 -- Breaker22/LConn3
  Three-Phase Measurement 1/LConn1 -- Three-Phase Measurement 4/RConn1
  Three-Phase Measurement 4/RConn2 -- Three-Phase Measurement 1/LConn2
  Three-Phase Measurement 4/RConn3 -- Three-Phase Measurement 1/LConn3
  Three-Phase RL Load20/LConn1 -- Breaker24/LConn1
  Three-Phase RL Load20/LConn3 -- Breaker24/LConn3
  Three-Phase RL Load19/LConn1 -- Breaker23/RConn1
  Three-Phase RL Load19/LConn3 -- Breaker23/RConn3
  Three-Phase RL Load20/LConn2 -- Breaker24/LConn2
  Three-Phase RL Load19/LConn2 -- Breaker23/RConn2
  Three-Phase Measurement 4/LConn3 -- Breaker21/RConn3 -- Breaker20/LConn3
  Three-Phase Measurement 4/LConn1 -- Breaker21/RConn1 -- Breaker20/LConn1
  Three-Phase Measurement 4/LConn2 -- Breaker21/RConn2 -- Breaker20/LConn2
  Three-Phase Transformer (Two Windings)2/LConn1 -- Breaker25/RConn1
  Three-Phase Transformer (Two Windings)2/LConn2 -- Breaker25/RConn2
  Three-Phase Transformer (Two Windings)2/LConn3 -- Breaker25/RConn3
  Breaker25/LConn1 -- Three-Phase V-I Measurement1/RConn1
  Breaker25/LConn2 -- Three-Phase V-I Measurement1/RConn2
  Breaker25/LConn3 -- Three-Phase V-I Measurement1/RConn3
  Three-Phase Transformer (Two Windings)1/LConn1 -- Breaker26/LConn1
  Three-Phase Transformer (Two Windings)1/LConn2 -- Breaker26/LConn2
  Three-Phase Transformer (Two Windings)1/LConn3 -- Breaker26/LConn3
  Breaker26/RConn1 -- Three-Phase V-I Measurement2/RConn1
  Breaker26/RConn2 -- Three-Phase V-I Measurement2/RConn2
  Breaker26/RConn3 -- Three-Phase V-I Measurement2/RConn3
  Series RLC Branch18/RConn1 -- Breaker19/LConn1
  Series RLC Branch18/LConn1 -- Breaker16/RConn1
  Series RLC Branch20/LConn1 -- Breaker16/RConn2
  Series RLC Branch19/LConn1 -- Breaker16/RConn3
  Series RLC Branch20/RConn1 -- Breaker19/LConn2
  Series RLC Branch19/RConn1 -- Breaker19/LConn3
  Series RLC Branch3/LConn1 -- Breaker21/LConn2
  Series RLC Branch2/LConn1 -- Breaker21/LConn3
  Series RLC Branch1/LConn1 -- Breaker21/LConn1
  Series RLC Branch1/RConn1 -- Breaker18/LConn1
  Series RLC Branch3/RConn1 -- Breaker18/LConn2
  Series RLC Branch2/RConn1 -- Breaker18/LConn3
  Series RLC Branch11/RConn1 -- Breaker29/RConn1 -- Series RLC Branch5/LConn1
  Series RLC Branch9/RConn1 -- Breaker29/RConn2 -- Series RLC Branch4/LConn1
  Series RLC Branch6/RConn1 -- Breaker29/RConn3 -- Series RLC Branch10/LConn1
  Three-Phase V-I Measurement4/LConn2 -- Three-Phase Series RLC Branch4/RConn2
  Three-Phase Series RLC Branch4/LConn2 -- Three-Phase Programmable Voltage Source4/RConn2
  Three-Phase Programmable Voltage Source4/LConn1 -- Ground3/LConn1
  Three-Phase Series RLC Branch4/RConn1 -- Three-Phase V-I Measurement4/LConn1
  Three-Phase Series RLC Branch4/RConn3 -- Three-Phase V-I Measurement4/LConn3
  Three-Phase Series RLC Branch4/LConn3 -- Three-Phase Programmable Voltage Source4/RConn3
  Three-Phase Series RLC Branch4/LConn1 -- Three-Phase Programmable Voltage Source4/RConn1
  Three-Phase V-I Measurement4/RConn1 -- Series RLC Branch7/LConn1
  Three-Phase V-I Measurement4/RConn2 -- Series RLC Branch21/LConn1
  Three-Phase V-I Measurement4/RConn3 -- Series RLC Branch8/LConn1
  Series RLC Branch7/RConn1 -- Breaker27/RConn1
  Series RLC Branch21/RConn1 -- Breaker27/RConn2
  Series RLC Branch8/RConn1 -- Breaker27/RConn3
  Series RLC Branch10/RConn1 -- Breaker17/RConn3
  Series RLC Branch5/RConn1 -- Breaker17/RConn1
  Series RLC Branch4/RConn1 -- Breaker17/RConn2
  Series RLC Branch6/LConn1 -- Breaker20/RConn3
  Series RLC Branch9/LConn1 -- Breaker20/RConn2
  Series RLC Branch11/LConn1 -- Breaker20/RConn1
  Breaker28/RConn3 -- Three-Phase Source1/RConn3
  Breaker28/LConn1 -- Three-Phase Measurement 9/LConn1
  Breaker28/RConn1 -- Three-Phase Source1/RConn1
  Three-Phase Measurement 9/RConn1 -- Series RLC Branch12/LConn1
  Breaker28/LConn2 -- Three-Phase Measurement 9/LConn2
  Breaker28/LConn3 -- Three-Phase Measurement 9/LConn3
  Breaker28/RConn2 -- Three-Phase Source1/RConn2
  Three-Phase Measurement 9/RConn3 -- Series RLC Branch13/LConn1
  Three-Phase Measurement 9/RConn2 -- Series RLC Branch14/LConn1
  Breaker29/LConn3 -- Series RLC Branch15/RConn1
  Series RLC Branch15/LConn1 -- Breaker31/RConn3
  Breaker31/LConn2 -- T1/RConn2
  Breaker29/LConn1 -- Series RLC Branch16/RConn1
  Breaker31/RConn1 -- Series RLC Branch16/LConn1
  Breaker29/LConn2 -- Series RLC Branch17/RConn1
  Breaker32/RConn1 -- Series RLC Branch23/LConn1
  Breaker31/LConn1 -- T1/RConn1
  Breaker32/LConn1 -- T1/RConn4
  Series RLC Branch22/LConn1 -- Breaker32/RConn3
  Breaker31/RConn2 -- Series RLC Branch17/LConn1
  Breaker30/RConn1 -- T1/LConn1
  Breaker30/RConn3 -- T1/LConn3
  Breaker32/LConn3 -- T1/RConn6
  Three-Phase RL Load21/LConn2 -- Series RLC Branch24/RConn1
  Breaker32/LConn2 -- T1/RConn5
  Three-Phase RL Load21/LConn3 -- Series RLC Branch22/RConn1
  Breaker31/LConn3 -- T1/RConn3
  Series RLC Branch24/LConn1 -- Breaker32/RConn2
  Three-Phase RL Load21/LConn1 -- Series RLC Branch23/RConn1
  Breaker30/RConn2 -- T1/LConn2
  Series RLC Branch12/RConn1 -- Breaker30/LConn1
  Series RLC Branch14/RConn1 -- Breaker30/LConn2
  Series RLC Branch13/RConn1 -- Breaker30/LConn3
  Breaker34/LConn2 -- Three-Phase V-I Measurement3/LConn2
  Three-Phase V-I Measurement3/RConn3 -- Breaker33/RConn3
  Three-Phase Fault/LConn3 -- Breaker33/LConn3
  Three-Phase V-I Measurement3/RConn2 -- Breaker33/RConn2
  Breaker33/LConn2 -- Three-Phase Fault/LConn2
  Three-Phase V-I Measurement3/LConn3 -- Breaker34/LConn3
  Breaker34/LConn1 -- Three-Phase V-I Measurement3/LConn1
  Three-Phase V-I Measurement3/RConn1 -- Breaker33/RConn1
  Breaker33/LConn1 -- Three-Phase Fault/LConn1
  Synchronous Machine/RConn2 -- Three-Phase Measurement 2/LConn2
  Synchronous Machine/RConn1 -- Three-Phase Measurement 2/LConn1
  Synchronous Machine/RConn3 -- Three-Phase Measurement 2/LConn3
